simulink model "problem12"  (R2021a)
settings: Solver=VariableStepAuto  StartTime=0.0  StopTime=10.0  RelTol=1e-3
undefined symbols (not defined in the file): Kd_1, Kd_2, Kd_3, Kd_4, Kp_1, Kp_2, Kp_3, Kp_4, qr_1, qr_2, qr_3, qr_4, T_L
settings Model: Creator=Luky  LastModifiedBy=Luky

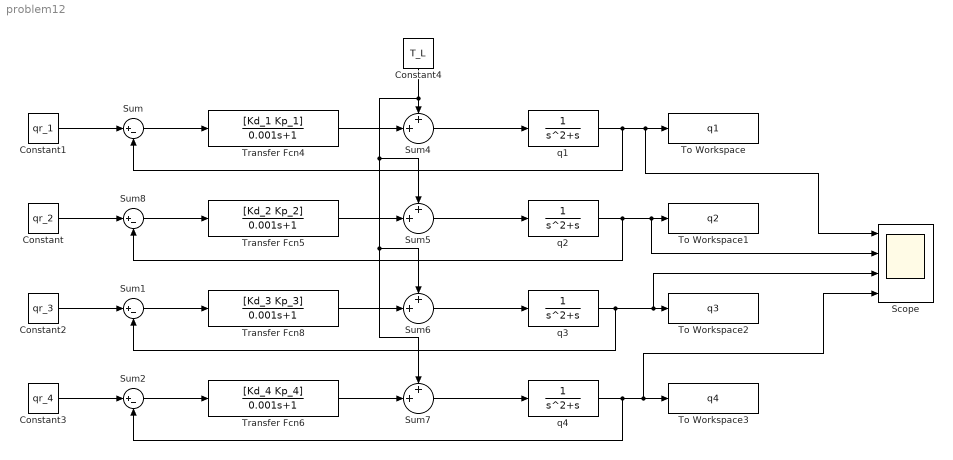
== system problem12 ==
  Constant : Constant  Value=qr_2
  Constant1 : Constant  Value=qr_1
  Constant2 : Constant  Value=qr_3
  Constant3 : Constant  Value=qr_4
  Constant4 : Constant  Value=T_L
  Scope : Scope  NumInputPorts=4
  Sum{,1..2,8} (4 alike) : Sum  Inputs=|+-
  Sum{4..7} (4 alike) : Sum  Inputs=++|
  To Workspace : ToWorkspace  VariableName=q1  SaveFormat=Timeseries  SampleTime=-1
  To Workspace1 : ToWorkspace  VariableName=q2  SaveFormat=Timeseries  SampleTime=-1
  To Workspace2 : ToWorkspace  VariableName=q3  SaveFormat=Timeseries  SampleTime=-1
  To Workspace3 : ToWorkspace  VariableName=q4  SaveFormat=Timeseries  SampleTime=-1
  Transfer Fcn4 : TransferFcn  Numerator=[Kd_1 Kp_1]  Denominator=[0.001 1]
  Transfer Fcn5 : TransferFcn  Numerator=[Kd_2 Kp_2]  Denominator=[0.001 1]
  Transfer Fcn6 : TransferFcn  Numerator=[Kd_4 Kp_4]  Denominator=[0.001 1]
  Transfer Fcn8 : TransferFcn  Numerator=[Kd_3 Kp_3]  Denominator=[0.001 1]
  q{1..4} (4 alike) : TransferFcn  Denominator=[1 1 0]
  wires:
  q1/1 -> Sum/2, Scope/1, To Workspace/1
  q2/1 -> Sum8/2, Scope/2, To Workspace1/1
  q3/1 -> Sum1/2, Scope/3, To Workspace2/1
  q4/1 -> Sum2/2, Scope/4, To Workspace3/1
  Sum/1 -> Transfer Fcn4/1
  Constant1/1 -> Sum/1
  Constant/1 -> Sum8/1
  Sum8/1 -> Transfer Fcn5/1
  Constant2/1 -> Sum1/1
  Sum1/1 -> Transfer Fcn8/1
  Constant3/1 -> Sum2/1
  Sum2/1 -> Transfer Fcn6/1
  Transfer Fcn4/1 -> Sum4/2
  Sum4/1 -> q1/1
  Sum6/1 -> q3/1
  Transfer Fcn5/1 -> Sum5/2
  Sum5/1 -> q2/1
  Sum7/1 -> q4/1
  Constant4/1 -> Sum7/1, Sum6/1, Sum5/1, Sum4/1
  Transfer Fcn8/1 -> Sum6/2
  Transfer Fcn6/1 -> Sum7/2
